simulink model "Q10"  (R2015a)
settings: Solver=ode45  StartTime=0.0  StopTime=10.0  RelTol=1e-3
values from neighbouring files (symbols this model uses):
  beta = 0.001    [lab3.m]
  cte3 = m*g*l + M*g*L/2    (= 0.4753)    [lab3.m]
  cte4 = 1/(((M*(L^2))/3 + m*(l^2)))    (= 60.6673407482)    [lab3.m]
  k = 0.35    [lab3.m]
  teta0 = pi/4    (= 0.785398163397)    [lab3.m]
  U = 0    [lab3.m]
  v0 = 0    [lab3.m]
settings Model: Creator=Diogo  LastModifiedBy=Diogo

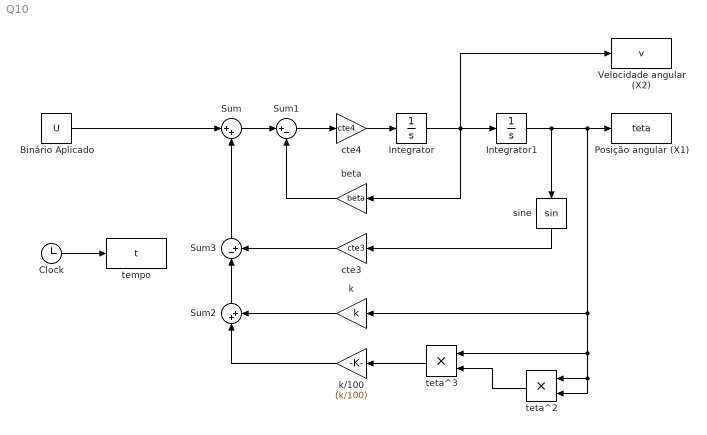
== system Q10 ==
  Binário Aplicado : Constant  Value=U
  Clock : Clock
  Integrator : Integrator  InitialCondition=v0
  Integrator1 : Integrator  InitialCondition=teta0
  Posição angular (X1) : ToWorkspace  VariableName=teta  SampleTime=0.001
  Sum : Sum  Inputs=|++
  Sum1 : Sum  Inputs=|+-
  Sum2 : Sum  Inputs=|++
  Sum3 : Sum  Inputs=|-+
  Velocidade angular (X2) : ToWorkspace  VariableName=v  SampleTime=0.001
  beta : Gain  Gain=beta
  cte3 : Gain  Gain=cte3
  cte4 : Gain  Gain=cte4
  k : Gain  Gain=k
  k/100 : Gain  Gain=(k/100)
  sine : Trigonometry
  tempo : ToWorkspace  VariableName=t  SampleTime=0.001
  "teta^2 " : Product
  teta^3 : Product
  wires:
  Binário Aplicado/1 -> Sum/1
  Integrator1/1 -> k/1, teta^3/1, "teta^2 "/1, "teta^2 "/2, Posição angular (X1)/1, sine/1
  Clock/1 -> tempo/1
  Integrator/1 -> Velocidade angular (X2)/1, beta/1, Integrator1/1
  sine/1 -> cte3/1
  "teta^2 "/1 -> teta^3/2
  teta^3/1 -> k/100/1
  cte3/1 -> Sum3/2
  Sum3/1 -> Sum/2
  cte4/1 -> Integrator/1
  beta/1 -> Sum1/2
  Sum1/1 -> cte4/1
  Sum/1 -> Sum1/1
  k/1 -> Sum2/2
  k/100/1 -> Sum2/1
  Sum2/1 -> Sum3/1
